simulink model "tarea_ejercicio3_02_02_17"  (R2013a)
settings: Solver=ode45  StartTime=0.0  StopTime=20  RelTol=1e-3
libraries: dspsrcs4 x2, simulink x2
settings Model: Creator=Miguel  LastModifiedBy=Miguel

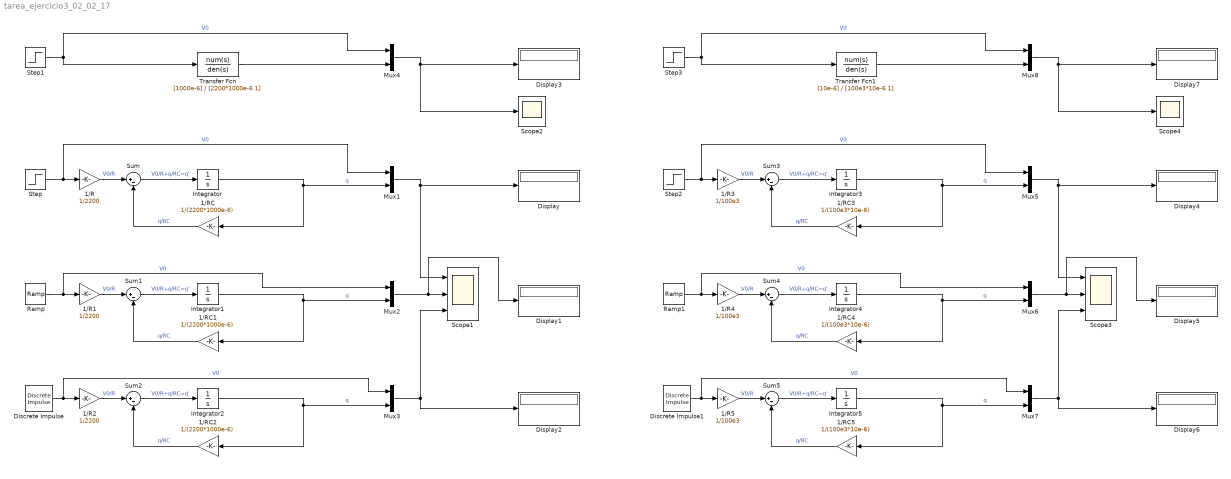
== system tarea_ejercicio3_02_02_17 ==
  1/R : Gain  Gain=1/2200
  1/R1 : Gain  Gain=1/2200
  1/R2 : Gain  Gain=1/2200
  1/R3 : Gain  Gain=1/100e3
  1/R4 : Gain  Gain=1/100e3
  1/R5 : Gain  Gain=1/100e3
  1/RC : Gain  Gain=1/(2200*1000e-6)
  1/RC1 : Gain  Gain=1/(2200*1000e-6)
  1/RC2 : Gain  Gain=1/(2200*1000e-6)
  1/RC3 : Gain  Gain=1/(100e3*10e-6)
  1/RC4 : Gain  Gain=1/(100e3*10e-6)
  1/RC5 : Gain  Gain=1/(100e3*10e-6)
  Discrete Impulse : dspsrcs4/Discrete  Impulse  Delay=0  SampleTime=1  FrameSample=1  dataType=double  isSigned=on  wordLen=16  udDataType=sfix(16)  fracBitsMode=Best precision  numFracBits=15  OutDataTypeStr=double  LastOutDataTypeStr=double
  Discrete Impulse1 : dspsrcs4/Discrete  Impulse  Delay=0  SampleTime=1  FrameSample=1  dataType=double  isSigned=on  wordLen=16  udDataType=sfix(16)  fracBitsMode=Best precision  numFracBits=15  OutDataTypeStr=double  LastOutDataTypeStr=double
  Display{,1..7} (8 alike) : Display
  Integrator{,1..5} (6 alike) : Integrator
  Mux{1..8} (8 alike) : Mux  Inputs=2
  Ramp : simulink/Sources/Ramp  slope=1  start=0  X0=0
  Ramp1 : simulink/Sources/Ramp  slope=1  start=0  X0=0
  Scope1 : Scope  NumInputPorts=3
      settings: TickLabels=on  ShowLegends=on  YMin=-5~-5~-5  YMax=5~5~5
  Scope2 : Scope
      settings: TickLabels=on  ShowLegends=on  TimeRange=20  YMin=0  YMax=1
  Scope3 : Scope  NumInputPorts=3
      settings: TickLabels=on  ShowLegends=on  YMin=-5~-5~-5  YMax=5~5~5  SaveName=ScopeData2
  Scope4 : Scope
      settings: TickLabels=on  ShowLegends=on  TimeRange=20  YMin=0  YMax=1  SaveName=ScopeData3
  Step{,1..3} (4 alike) : Step  SampleTime=0
  Sum{,1..5} (6 alike) : Sum  Inputs=|+-
  Transfer Fcn : TransferFcn  Numerator=[1000e-6]  Denominator=[2200*1000e-6 1]
  Transfer Fcn1 : TransferFcn  Numerator=[10e-6]  Denominator=[100e3*10e-6 1]
  wires:
  Mux2/1 -> Display1/1, Scope1/2
  Mux1/1 -> Display/1, Scope1/1
  Mux3/1 -> Display2/1, Scope1/3
  Step/1 -> Mux1/1, 1/R/1  "V0"
  1/R/1 -> Sum/1  "V0/R"
  Sum/1 -> Integrator/1  "V0/R+q/RC=q'"
  Integrator/1 -> Mux1/2, 1/RC/1  "q"
  1/RC/1 -> Sum/2  "q/RC"
  Ramp/1 -> Mux2/1, 1/R1/1  "V0"
  1/R1/1 -> Sum1/1  "V0/R"
  Sum1/1 -> Integrator1/1  "V0/R+q/RC=q'"
  Integrator1/1 -> Mux2/2, 1/RC1/1  "q"
  1/RC1/1 -> Sum1/2  "q/RC"
  Discrete Impulse/1 -> Mux3/1, 1/R2/1  "V0"
  1/R2/1 -> Sum2/1  "V0/R"
  Sum2/1 -> Integrator2/1  "V0/R+q/RC=q'"
  Integrator2/1 -> Mux3/2, 1/RC2/1  "q"
  1/RC2/1 -> Sum2/2  "q/RC"
  Mux4/1 -> Display3/1, Scope2/1
  Step1/1 -> Mux4/1, Transfer Fcn/1  "V0"
  Transfer Fcn/1 -> Mux4/2
  Mux6/1 -> Display5/1, Scope3/2
  Mux5/1 -> Display4/1, Scope3/1
  Mux7/1 -> Display6/1, Scope3/3
  Step2/1 -> Mux5/1, 1/R3/1  "V0"
  1/R3/1 -> Sum3/1  "V0/R"
  Sum3/1 -> Integrator3/1  "V0/R+q/RC=q'"
  Integrator3/1 -> Mux5/2, 1/RC3/1  "q"
  1/RC3/1 -> Sum3/2  "q/RC"
  Ramp1/1 -> Mux6/1, 1/R4/1  "V0"
  1/R4/1 -> Sum4/1  "V0/R"
  Sum4/1 -> Integrator4/1  "V0/R+q/RC=q'"
  Integrator4/1 -> Mux6/2, 1/RC4/1  "q"
  1/RC4/1 -> Sum4/2  "q/RC"
  Discrete Impulse1/1 -> Mux7/1, 1/R5/1  "V0"
  1/R5/1 -> Sum5/1  "V0/R"
  Sum5/1 -> Integrator5/1  "V0/R+q/RC=q'"
  Integrator5/1 -> Mux7/2, 1/RC5/1  "q"
  1/RC5/1 -> Sum5/2  "q/RC"
  Mux8/1 -> Display7/1, Scope4/1
  Step3/1 -> Mux8/1, Transfer Fcn1/1  "V0"
  Transfer Fcn1/1 -> Mux8/2
